simulink model "processor_with_peripherals"  (R2025a)
settings: Solver=FixedStepDiscrete  StartTime=0.0  StopTime=inf  RelTol=1e-3
libraries: simulink x6
(part 4 of 5)

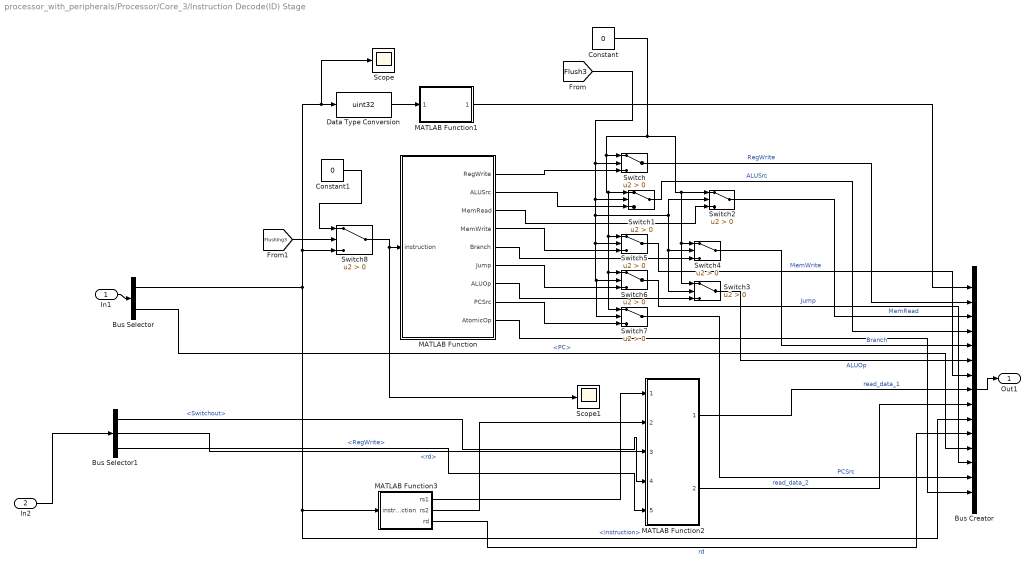
== system processor_with_peripherals/Processor/Core_3/Instruction Decode(ID) Stage ==
  In1 : Inport
  In2 : Inport  Port=2
  Bus Creator : BusCreator  Inputs=15  OutDataTypeStr=Bus: IDEX_Bus  NonVirtualBus=on
  Bus Selector : BusSelector  OutputSignals=Instruction,PC
  Bus Selector1 : BusSelector  OutputSignals=Switchout,rd,RegWrite
  Constant : Constant  Value=0  OutDataTypeStr=uint8
  Constant1 : Constant  Value=0
  Data Type Conversion : DataTypeConversion  OutDataTypeStr=uint32  SaturateOnIntegerOverflow=off  RndMeth=Floor
  MATLAB Function : MATLAB Function  TreatAsAtomicUnit=on
  MATLAB Function1 : MATLAB Function  TreatAsAtomicUnit=on
  MATLAB Function2 : MATLAB Function  TreatAsAtomicUnit=on
  MATLAB Function3 : MATLAB Function  TreatAsAtomicUnit=on
  Scope : Scope
      settings: ActiveDisplayYMinimum=-8.6059552101299882E+7  ActiveDisplayYMaximum=2.8669047582629967E+8  DataLoggingVariableName=ScopeData4
  Scope1 : Scope
      settings: ActiveDisplayYMinimum=-0.20992987297977578  ActiveDisplayYMaximum=4.3440753791982463  DataLoggingVariableName=ScopeData5
  Switch{,1..2,5..6} (5 alike) : Switch  Criteria=u2 > Threshold  OutDataTypeStr=boolean  SaturateOnIntegerOverflow=off  InputSameDT=off
  Switch3 : Switch  Criteria=u2 > Threshold  OutDataTypeStr=uint32  SaturateOnIntegerOverflow=off  InputSameDT=off
  Switch4 : Switch  Criteria=u2 > Threshold  OutDataTypeStr=uint32  SaturateOnIntegerOverflow=off  InputSameDT=off
  Switch7 : Switch  Criteria=u2 > Threshold  OutDataTypeStr=uint32  SaturateOnIntegerOverflow=off  InputSameDT=off
  Switch8 : Switch  Criteria=u2 > Threshold  SaturateOnIntegerOverflow=off  InputSameDT=off
  Out1 : Outport
  wires:
  Bus Creator/1 -> Out1/1
  In1/1 -> Bus Selector/1
  Bus Selector/1 -> Data Type Conversion/1, Scope/1, Switch8/3, MATLAB Function3/1(instruction), Bus Creator/10  "<Instruction>"
  MATLAB Function2/1(ReadData1) -> Bus Creator/8  "read_data_1"
  MATLAB Function2/2(ReadData2) -> Bus Creator/9  "read_data_2"
  MATLAB Function1/1(immediate_out) -> Bus Creator/1
  MATLAB Function3/3(rd) -> Bus Creator/11  "rd"
  MATLAB Function/7(ALUOp) -> Switch3/3
  MATLAB Function/6(Jump) -> Switch6/3
  MATLAB Function/5(Branch) -> Switch4/3
  MATLAB Function/4(MemWrite) -> Switch5/3
  MATLAB Function/3(MemRead) -> Switch2/3
  MATLAB Function/2(ALUSrc) -> Switch1/3
  Bus Selector1/2 -> MATLAB Function2/3(WriteAddr)  "<rd>"
  Bus Selector1/3 -> MATLAB Function2/5(WriteEnable)  "<RegWrite>"
  Bus Selector1/1 -> MATLAB Function2/4(WriteData)  "<Switchout>"
  MATLAB Function3/2(rs2) -> MATLAB Function2/2(ReadAddr2)
  Bus Selector/2 -> Bus Creator/12  "<PC>"
  MATLAB Function/8(PCSrc) -> Switch7/3
  MATLAB Function/1(RegWrite) -> Switch/3
  [Flush3] -> Switch1/2, Switch3/2, Switch4/2, Switch2/2, Switch7/2, Switch6/2, Switch5/2, Switch/2
  Constant/1 -> Switch3/1, Switch4/1, Switch2/1, Switch7/1, Switch6/1, Switch5/1, Switch1/1, Switch/1
  Switch/1 -> Bus Creator/2  "RegWrite"
  Switch2/1 -> Bus Creator/3  "MemRead"
  Switch1/1 -> Bus Creator/4  "ALUSrc"
  Switch4/1 -> Bus Creator/5  "Branch"
  Switch3/1 -> Bus Creator/6  "ALUOp"
  Switch5/1 -> Bus Creator/7  "MemWrite"
  Switch6/1 -> Bus Creator/13  "Jump"
  Switch7/1 -> Bus Creator/14  "PCSrc"
  MATLAB Function3/1(rs1) -> MATLAB Function2/1(ReadAddr1)
  In2/1 -> Bus Selector1/1
  Switch8/1 -> Scope1/1, MATLAB Function/1(instruction)
  Constant1/1 -> Switch8/1
  [Flushing3] -> Switch8/2
  Data Type Conversion/1 -> MATLAB Function1/1(instruction)
  MATLAB Function/9(AtomicOp) -> Bus Creator/15

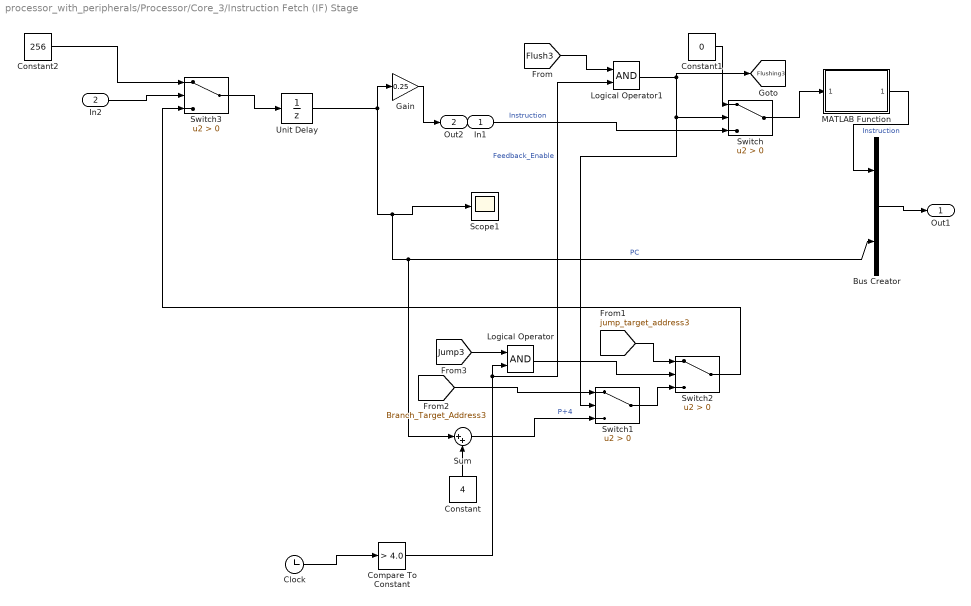
== system processor_with_peripherals/Processor/Core_3/Instruction Fetch (IF) Stage ==
  In1 : Inport
  In2 : Inport  Port=2
  Bus Creator : BusCreator  Inputs=2  OutDataTypeStr=Bus: IFID_Bus  NonVirtualBus=on
  Clock : Clock
  Compare To Constant : simulink/Logic and Bit Operations/Compare To Constant  relop=>  const=4.0  OutDataTypeStr=boolean
  Constant : Constant  Value=4
  Constant1 : Constant  Value=0
  Constant2 : Constant  Value=256  OutDataTypeStr=uint32
  Gain : Gain  Gain=0.25  OutDataTypeStr=uint32
  Logical Operator : Logic  AllPortsSameDT=off  OutDataTypeStr=boolean
  Logical Operator1 : Logic  AllPortsSameDT=off  OutDataTypeStr=boolean
  MATLAB Function : MATLAB Function  TreatAsAtomicUnit=on
  Scope1 : Scope
      settings: ActiveDisplayYMinimum=14.083038013644533  ActiveDisplayYMaximum=56.284353840527714  DataLoggingVariableName=ScopeData6
  Sum : Sum  Inputs=|++  OutDataTypeStr=uint32  AccumDataTypeStr=uint32
  Switch : Switch  Criteria=u2 > Threshold  OutDataTypeStr=uint32  SaturateOnIntegerOverflow=off  InputSameDT=off
  Switch1 : Switch  Criteria=u2 > Threshold  OutDataTypeStr=uint32  SaturateOnIntegerOverflow=off  InputSameDT=off
  Switch2 : Switch  Criteria=u2 > Threshold  OutDataTypeStr=uint32  SaturateOnIntegerOverflow=off  InputSameDT=off
  Switch3 : Switch  Criteria=u2 > Threshold  SaturateOnIntegerOverflow=off  InputSameDT=off
  Unit Delay : UnitDelay  HasFrameUpgradeWarning=on
  Out1 : Outport
  Out2 : Outport  Port=2
  tag scope: Flushing3=global
  wires:
  Unit Delay/1 -> Scope1/1, Bus Creator/2, Sum/1, Gain/1  "PC"
  Constant/1 -> Sum/2
  In1/1 -> Switch/3  "Instruction"
  [jump_target_address3] -> Switch2/1
  Logical Operator1/1 -> Switch/2, Switch1/2, [Flushing3]
  Sum/1 -> Switch1/3  "P+4"
  Bus Creator/1 -> Out1/1
  Switch1/1 -> Switch2/3
  Switch2/1 -> Switch3/3
  [Jump3] -> Logical Operator/1
  [Branch_Target_Address3] -> Switch1/1
  Clock/1 -> Compare To Constant/1
  Compare To Constant/1 -> Logical Operator1/2, Logical Operator/2  "Feedback_Enable"
  Logical Operator/1 -> Switch2/2
  [Flush3] -> Logical Operator1/1
  MATLAB Function/1(scalar_out) -> Bus Creator/1  "Instruction"
  Switch/1 -> MATLAB Function/1(vector_in)
  Constant1/1 -> Switch/1
  Gain/1 -> Out2/1
  Switch3/1 -> Unit Delay/1
  In2/1 -> Switch3/2
  Constant2/1 -> Switch3/1

== system processor_with_peripherals/Processor/Core_3/Memory Access ==
  In1 : Inport
  Bus Creator : BusCreator  Inputs=4  OutDataTypeStr=Bus: MEMWB_Bus
  Bus Selector : BusSelector  OutputSignals=read_data_2,ALU_Result,MemWrite,RegWrite,MemRead,rd,AtomicOp
  Switch : Switch  Criteria=u2 > Threshold  SaturateOnIntegerOverflow=off  InputSameDT=off
  Out1 : Outport
  Out2 : Outport  Port=2
  Out3 : Outport  Port=3
  Out4 : Outport  Port=4
  Out5 : Outport  Port=5
  wires:
  In1/1 -> Bus Selector/1
  Bus Selector/2 -> Switch/1, Out2/1, Bus Creator/1  "<ALU_Result>"
  Bus Selector/6 -> Bus Creator/4  "<rd>"
  Bus Selector/3 -> Out5/1  "<MemWrite>"
  Bus Selector/5 -> Bus Creator/3, Out4/1  "<MemRead>"
  Bus Selector/4 -> Bus Creator/2  "<RegWrite>"
  Bus Selector/1 -> Switch/3  "<read_data_2>"
  Bus Creator/1 -> Out1/1
  Switch/1 -> Out3/1
  Bus Selector/7 -> Switch/2  "<AtomicOp>"

== system processor_with_peripherals/Processor/Core_3/Write Back ==
  In1 : Inport
  In2 : Inport  Port=2
  Bus Creator : BusCreator  Inputs=3
  Bus Selector : BusSelector  OutputSignals=ALU_Result,rd,MemRead,RegWrite
  Switch : Switch  Criteria=u2 > Threshold  SaturateOnIntegerOverflow=off  InputSameDT=off
  Out1 : Outport
  wires:
  Bus Creator/1 -> Out1/1
  In1/1 -> Bus Selector/1
  Bus Selector/1 -> Switch/3  "<ALU_Result>"
  Bus Selector/2 -> Bus Creator/2  "<rd>"
  Bus Selector/4 -> Bus Creator/3  "<RegWrite>"
  Bus Selector/3 -> Switch/2  "<MemRead>"
  Switch/1 -> Bus Creator/1  "Switchout"
  In2/1 -> Switch/1

== matlab function processor_with_peripherals/Processor/Core_2/Execute (EX) Stage/MATLAB Function ==
  data: Operand1 input; ALU_Result output int32 size=1; Operand2 input; ALUOp input; Instruction input; Zero_Flag output boolean size=1; AtomicOp input
function [ALU_Result, Zero_Flag] = alu(Operand1, Operand2, ALUOp, Instruction, AtomicOp)
% This is the final ALU code, supporting standard operations and
% the RISC-V "A" extension for atomic memory operations.

    instr = uint32(Instruction);
    alu_op_val = ALUOp(1)*2 + ALUOp(2); 

    % Extract function fields
    funct3 = bitshift(bitand(instr, uint32(hex2dec('7000'))), -12);
    funct7 = bitshift(bitand(instr, uint32(hex2dec('FE000000'))), -25);
    funct5 = bitshift(bitand(instr, uint32(hex2dec('F8000000'))), -27); % For atomic ops

    ALU_Result = int32(0);

    if AtomicOp
        % --- This is an Atomic Operation ---
        switch funct5
            case 0,  ALU_Result = Operand1 + Operand2;  % AMOADD.W
            case 1,  ALU_Result = Operand2;            % AMOSWAP.W
            case 4,  ALU_Result = bitxor(Operand1, Operand2); % AMOXOR.W
            case 12, ALU_Result = bitand(Operand1, Operand2); % AMOAND.W
            case 20, ALU_Result = bitor(Operand1, Operand2);  % AMOOR.W
            otherwise, ALU_Result = Operand1;
        end
    else
        % --- This is a Normal Operation ---
        switch alu_op_val
            case 0 % For LW, SW, ADDI, JAL, etc.
                ALU_Result = Operand1 + Operand2;
            case 1 % For Branches
                ALU_Result = Operand1 - Operand2;
            case 2 % R-type instructions
                switch funct3
                    case 0 % ADD or SUB
                        if funct7 == 32, ALU_Result = Operand1 - Operand2; else, ALU_Result = Operand1 + Operand2; end
                    case 1, ALU_Result = int32(bitshift(uint32(Operand1), Operand2)); % SLL
                    case 2, if Operand1 < Operand2, ALU_Result = int32(1); else, ALU_Result = int32(0); end % SLT
                    case 4, ALU_Result = bitxor(Operand1, Operand2); % XOR
                    case 6, ALU_Result = bitor(Operand1, Operand2);  % OR
                    case 7, ALU_Result = bitand(Operand1, Operand2); % AND
                    otherwise, ALU_Result = int32(0);
                end
            case 3 % I-type instructions
                 switch funct3
                    case 0, ALU_Result = Operand1 + Operand2; % ADDI
                    case 2, if Operand1 < Operand2, ALU_Result = int32(1); else, ALU_Result = int32(0); end % SLTI
                    case 4, ALU_Result = bitxor(Operand1, Operand2); % XORI
                    case 6, ALU_Result = bitor(Operand1, Operand2);  % ORI
                    case 7, ALU_Result = bitand(Operand1, Operand2); % ANDI
                    otherwise, ALU_Result = int32(0);
                 end
        end
    end
    
    Zero_Flag = (ALU_Result == 0);
end

== matlab function processor_with_peripherals/Processor/Core_1/Instruction Decode(ID) Stage/MATLAB Function ==
  data: instruction input; RegWrite output; ALUSrc output; MemRead output; MemWrite output; Branch output; Jump output boolean; ALUOp output; PCSrc output; AtomicOp output
function [RegWrite, ALUSrc, MemRead, MemWrite, Branch, Jump, ALUOp, PCSrc, AtomicOp] = control_unit(instruction)
% This is the final Control Unit code. It takes an instruction and
% generates all necessary control signals for the datapath.

    instr = uint32(instruction);
    
    % --- Opcode Definitions ---
    OPCODE_R_TYPE   = uint32(hex2dec('33'));
    OPCODE_I_TYPE   = uint32(hex2dec('13'));
    OPCODE_LOAD     = uint32(hex2dec('03'));
    OPCODE_STORE    = uint32(hex2dec('23'));
    OPCODE_BRANCH   = uint32(hex2dec('63'));
    OPCODE_JAL      = uint32(hex2dec('6F'));
    OPCODE_JALR     = uint32(hex2dec('67'));
    OPCODE_LUI      = uint32(hex2dec('37'));
    OPCODE_AMO      = uint32(hex2dec('2F'));

    % --- Control Signal Initialization ---
    RegWrite = false; ALUSrc = false; MemRead = false; MemWrite = false;
    Branch = false; Jump = false; PCSrc = false; AtomicOp = false;
    ALUOp = [0 0];
    
    opcode = bitand(instr, uint32(127));

    % --- Decoder Logic ---
    switch opcode
        case OPCODE_R_TYPE
            RegWrite = true; ALUSrc = false; ALUOp = [1 0];
        case OPCODE_I_TYPE
            RegWrite = true; ALUSrc = true; ALUOp = [1 1];
        case OPCODE_LOAD
            RegWrite = true; ALUSrc = true; MemRead = true; ALUOp = [0 0];
        case OPCODE_STORE
            ALUSrc = true; MemWrite = true; ALUOp = [0 0];
        case OPCODE_BRANCH
            Branch = true; ALUSrc = false; ALUOp = [0 1];
        case OPCODE_JAL
            RegWrite = true; Jump = true; ALUSrc = true; PCSrc = true; ALUOp = [0 0];
        case OPCODE_JALR
            RegWrite = true; Jump = true; ALUSrc = true; ALUOp = [0 0];
        case OPCODE_LUI
            RegWrite = true; ALUSrc = true; PCSrc = true; ALUOp = [0 0];
        case OPCODE_AMO
            RegWrite = true; MemRead = true; MemWrite = true; AtomicOp = true; ALUOp = [1 0];
    end
end

== matlab function processor_with_peripherals/Processor/Core_1/Instruction Decode(ID) Stage/MATLAB Function1 ==
  data: instruction input uint32; immediate_out output int32
function immediate_out = immediate_generator(instruction)
% This function uses a robust subtraction method for sign extension
% to prevent all overflow errors in the Simulink Coder.

    instr = uint32(instruction);
    opcode = bitand(instr, uint32(127));

    % Define opcodes
    OPCODE_I_TYPE   = uint32(hex2dec('13'));
    OPCODE_LOAD     = uint32(hex2dec('03'));
    OPCODE_JALR     = uint32(hex2dec('67'));
    OPCODE_STORE    = uint32(hex2dec('23'));
    OPCODE_BRANCH   = uint32(hex2dec('63'));
    OPCODE_LUI      = uint32(hex2dec('37'));
    OPCODE_JAL      = uint32(hex2dec('6F'));

    imm_val = int32(0); % Use a signed integer for the final value
    
    switch opcode
        case {OPCODE_I_TYPE, OPCODE_LOAD, OPCODE_JALR} % I-type
            imm_unsigned = bitshift(instr, -20);
            sign_bit = bitget(imm_unsigned, 12);
            if sign_bit
                % Two's complement: val - 2^12
                imm_val = int32(imm_unsigned) - 4096; 
            else
                imm_val = int32(imm_unsigned);
            end

        case OPCODE_STORE % S-type
            imm_11_5 = bitshift(instr, -25);
            imm_4_0  = bitshift(bitand(instr, uint32(hex2dec('F80'))), -7);
            imm_unsigned = bitor(imm_11_5, imm_4_0);
            sign_bit = bitget(imm_unsigned, 12);
            if sign_bit
                imm_val = int32(imm_unsigned) - 4096;
            else
                imm_val = int32(imm_unsigned);
            end
            
        case OPCODE_BRANCH % B-type
            imm_12   = bitshift(bitand(instr, uint32(hex2dec('80000000'))), -19);
            imm_10_5 = bitshift(bitand(instr, uint32(hex2dec('7E000000'))), -20);
            imm_4_1  = bitshift(bitand(instr, uint32(hex2dec('F00'))), -7);
            imm_11   = bitshift(bitand(instr, uint32(hex2dec('80'))), 4);
            imm_unsigned = bitor(bitor(bitor(imm_12, imm_11), imm_10_5), imm_4_1);
            sign_bit = bitget(imm_unsigned, 13);
            if sign_bit
                imm_val = int32(imm_unsigned) - 8192; % 2^13
            else
                imm_val = int32(imm_unsigned);
            end
        
        case OPCODE_LUI % U-type -- THIS IS THE FIX --
            % For LUI, the immediate is the entire upper 20 bits.
            % The value is simply the instruction bits themselves, treated
            % as a 32-bit signed number. We cast the uint32 instruction
            % directly to int32, which correctly interprets the sign bit.
            imm_val = typecast(instr, 'int32');

        case OPCODE_JAL % J-type
            imm_20   = bitshift(bitand(instr, uint32(hex2dec('80000000'))), -11);
            imm_10_1 = bitshift(bitand(instr, uint32(hex2dec('7FE00000'))), -20);
            imm_11   = bitshift(bitand(instr, uint32(hex2dec('100000'))), -9);
            imm_19_12= bitand(instr, uint32(hex2dec('FF000')));
            imm_unsigned = bitor(bitor(bitor(imm_20, imm_19_12), imm_11), imm_10_1);
            sign_bit = bitget(imm_unsigned, 21);
            if sign_bit
                imm_val = int32(imm_unsigned) - 2097152; % 2^21
            else
                imm_val = int32(imm_unsigned);
            end
    end
    
    immediate_out = imm_val;
end

== matlab function processor_with_peripherals/Processor/Core_1/Instruction Decode(ID) Stage/MATLAB Function2 ==
  data: ReadAddr1 input; ReadData1 output int32; ReadAddr2 input; WriteAddr input; WriteData input; WriteEnable input; ReadData2 output int32
function [ReadData1, ReadData2] = register_file(ReadAddr1, ReadAddr2, WriteAddr, WriteData, WriteEnable)
% Implements a 32-register file for a RISC-V processor.
% x0 is hardwired to zero. Uses 1-based MATLAB indexing.

    persistent Registers;
    if isempty(Registers)
        Registers = zeros(32, 1, 'int32');
    end

    % 1. Handle the Write-Back from the WB stage first (synchronous write)
    if WriteEnable
        if WriteAddr > 0 % Do not write to register x0
            % MATLAB arrays are 1-based, so we add 1 to the 0-based RISC-V address
            Registers(WriteAddr + 1) = WriteData;
        end
    end

    % 2. Perform the Reads for the ID stage (combinational read)
    if ReadAddr1 == 0
        ReadData1 = int32(0);
    else
        ReadData1 = Registers(ReadAddr1 + 1);
    end

    if ReadAddr2 == 0
        ReadData2 = int32(0);
    else
        ReadData2 = Registers(ReadAddr2 + 1);
    end
end

== matlab function processor_with_peripherals/Processor/Core_1/Instruction Decode(ID) Stage/MATLAB Function3 ==
  data: instruction input; rs1 output uint8; rs2 output uint8; rd output uint8
function [rs1, rs2, rd] = bit_slicer(instruction)
% This function correctly extracts the rs1, rs2, and rd fields
% from a 32-bit RISC-V instruction word.

    instr = uint32(instruction);

    % Extract rd (destination register, bits 11:7)
    rd  = uint8(bitshift(bitand(instr, uint32(hex2dec('F80'))), -7));

    % Extract rs1 (source register 1, bits 19:15)
    rs1 = uint8(bitshift(bitand(instr, uint32(hex2dec('F8000'))), -15));

    % Extract rs2 (source register 2, bits 24:20)
    rs2 = uint8(bitshift(bitand(instr, uint32(hex2dec('1F00000'))), -20));
end

== matlab function processor_with_peripherals/Processor/Core_1/Instruction Fetch (IF) Stage/MATLAB Function ==
  data: vector_in input; scalar_out output uint32
function scalar_out = to_scalar(vector_in)
% This function extracts the first element from an input vector
% and ensures the output is a uint32 scalar.
    scalar_out = uint32(vector_in(1));
end

== matlab function processor_with_peripherals/Processor/Core_2/Instruction Decode(ID) Stage/MATLAB Function ==
  data: instruction input; RegWrite output; ALUSrc output; MemRead output; MemWrite output; Branch output; Jump output boolean; ALUOp output; PCSrc output; AtomicOp output
function [RegWrite, ALUSrc, MemRead, MemWrite, Branch, Jump, ALUOp, PCSrc, AtomicOp] = control_unit(instruction)
% This is the final Control Unit code. It takes an instruction and
% generates all necessary control signals for the datapath.

    instr = uint32(instruction);
    
    % --- Opcode Definitions ---
    OPCODE_R_TYPE   = uint32(hex2dec('33'));
    OPCODE_I_TYPE   = uint32(hex2dec('13'));
    OPCODE_LOAD     = uint32(hex2dec('03'));
    OPCODE_STORE    = uint32(hex2dec('23'));
    OPCODE_BRANCH   = uint32(hex2dec('63'));
    OPCODE_JAL      = uint32(hex2dec('6F'));
    OPCODE_JALR     = uint32(hex2dec('67'));
    OPCODE_LUI      = uint32(hex2dec('37'));
    OPCODE_AMO      = uint32(hex2dec('2F'));

    % --- Control Signal Initialization ---
    RegWrite = false; ALUSrc = false; MemRead = false; MemWrite = false;
    Branch = false; Jump = false; PCSrc = false; AtomicOp = false;
    ALUOp = [0 0];
    
    opcode = bitand(instr, uint32(127));

    % --- Decoder Logic ---
    switch opcode
        case OPCODE_R_TYPE
            RegWrite = true; ALUSrc = false; ALUOp = [1 0];
        case OPCODE_I_TYPE
            RegWrite = true; ALUSrc = true; ALUOp = [1 1];
        case OPCODE_LOAD
            RegWrite = true; ALUSrc = true; MemRead = true; ALUOp = [0 0];
        case OPCODE_STORE
            ALUSrc = true; MemWrite = true; ALUOp = [0 0];
        case OPCODE_BRANCH
            Branch = true; ALUSrc = false; ALUOp = [0 1];
        case OPCODE_JAL
            RegWrite = true; Jump = true; ALUSrc = true; PCSrc = true; ALUOp = [0 0];
        case OPCODE_JALR
            RegWrite = true; Jump = true; ALUSrc = true; ALUOp = [0 0];
        case OPCODE_LUI
            RegWrite = true; ALUSrc = true; PCSrc = true; ALUOp = [0 0];
        case OPCODE_AMO
            RegWrite = true; MemRead = true; MemWrite = true; AtomicOp = true; ALUOp = [1 0];
    end
end

== matlab function processor_with_peripherals/Processor/Core_2/Instruction Decode(ID) Stage/MATLAB Function1 ==
  data: instruction input uint32; immediate_out output int32
function immediate_out = immediate_generator(instruction)
% This function uses a robust subtraction method for sign extension
% to prevent all overflow errors in the Simulink Coder.

    instr = uint32(instruction);
    opcode = bitand(instr, uint32(127));

    % Define opcodes
    OPCODE_I_TYPE   = uint32(hex2dec('13'));
    OPCODE_LOAD     = uint32(hex2dec('03'));
    OPCODE_JALR     = uint32(hex2dec('67'));
    OPCODE_STORE    = uint32(hex2dec('23'));
    OPCODE_BRANCH   = uint32(hex2dec('63'));
    OPCODE_LUI      = uint32(hex2dec('37'));
    OPCODE_JAL      = uint32(hex2dec('6F'));

    imm_val = int32(0); % Use a signed integer for the final value
    
    switch opcode
        case {OPCODE_I_TYPE, OPCODE_LOAD, OPCODE_JALR} % I-type
            imm_unsigned = bitshift(instr, -20);
            sign_bit = bitget(imm_unsigned, 12);
            if sign_bit
                % Two's complement: val - 2^12
                imm_val = int32(imm_unsigned) - 4096; 
            else
                imm_val = int32(imm_unsigned);
            end

        case OPCODE_STORE % S-type
            imm_11_5 = bitshift(instr, -25);
            imm_4_0  = bitshift(bitand(instr, uint32(hex2dec('F80'))), -7);
            imm_unsigned = bitor(imm_11_5, imm_4_0);
            sign_bit = bitget(imm_unsigned, 12);
            if sign_bit
                imm_val = int32(imm_unsigned) - 4096;
            else
                imm_val = int32(imm_unsigned);
            end
            
        case OPCODE_BRANCH % B-type
            imm_12   = bitshift(bitand(instr, uint32(hex2dec('80000000'))), -19);
            imm_10_5 = bitshift(bitand(instr, uint32(hex2dec('7E000000'))), -20);
            imm_4_1  = bitshift(bitand(instr, uint32(hex2dec('F00'))), -7);
            imm_11   = bitshift(bitand(instr, uint32(hex2dec('80'))), 4);
            imm_unsigned = bitor(bitor(bitor(imm_12, imm_11), imm_10_5), imm_4_1);
            sign_bit = bitget(imm_unsigned, 13);
            if sign_bit
                imm_val = int32(imm_unsigned) - 8192; % 2^13
            else
                imm_val = int32(imm_unsigned);
            end
        
        case OPCODE_LUI % U-type -- THIS IS THE FIX --
            % For LUI, the immediate is the entire upper 20 bits.
            % The value is simply the instruction bits themselves, treated
            % as a 32-bit signed number. We cast the uint32 instruction
            % directly to int32, which correctly interprets the sign bit.
            imm_val = typecast(instr, 'int32');

        case OPCODE_JAL % J-type
            imm_20   = bitshift(bitand(instr, uint32(hex2dec('80000000'))), -11);
            imm_10_1 = bitshift(bitand(instr, uint32(hex2dec('7FE00000'))), -20);
            imm_11   = bitshift(bitand(instr, uint32(hex2dec('100000'))), -9);
            imm_19_12= bitand(instr, uint32(hex2dec('FF000')));
            imm_unsigned = bitor(bitor(bitor(imm_20, imm_19_12), imm_11), imm_10_1);
            sign_bit = bitget(imm_unsigned, 21);
            if sign_bit
                imm_val = int32(imm_unsigned) - 2097152; % 2^21
            else
                imm_val = int32(imm_unsigned);
            end
    end
    
    immediate_out = imm_val;
end

== matlab function processor_with_peripherals/Processor/Core_2/Instruction Decode(ID) Stage/MATLAB Function2 ==
  data: ReadAddr1 input; ReadData1 output int32; ReadAddr2 input; WriteAddr input; WriteData input; WriteEnable input; ReadData2 output int32
function [ReadData1, ReadData2] = register_file(ReadAddr1, ReadAddr2, WriteAddr, WriteData, WriteEnable)
% Implements a 32-register file for a RISC-V processor.
% x0 is hardwired to zero. Uses 1-based MATLAB indexing.

    persistent Registers;
    if isempty(Registers)
        Registers = zeros(32, 1, 'int32');
    end

    % 1. Handle the Write-Back from the WB stage first (synchronous write)
    if WriteEnable
        if WriteAddr > 0 % Do not write to register x0
            % MATLAB arrays are 1-based, so we add 1 to the 0-based RISC-V address
            Registers(WriteAddr + 1) = WriteData;
        end
    end

    % 2. Perform the Reads for the ID stage (combinational read)
    if ReadAddr1 == 0
        ReadData1 = int32(0);
    else
        ReadData1 = Registers(ReadAddr1 + 1);
    end

    if ReadAddr2 == 0
        ReadData2 = int32(0);
    else
        ReadData2 = Registers(ReadAddr2 + 1);
    end
end

== matlab function processor_with_peripherals/Processor/Core_2/Instruction Decode(ID) Stage/MATLAB Function3 ==
  data: instruction input; rs1 output uint8; rs2 output uint8; rd output uint8
function [rs1, rs2, rd] = bit_slicer(instruction)
% This function correctly extracts the rs1, rs2, and rd fields
% from a 32-bit RISC-V instruction word.

    instr = uint32(instruction);

    % Extract rd (destination register, bits 11:7)
    rd  = uint8(bitshift(bitand(instr, uint32(hex2dec('F80'))), -7));

    % Extract rs1 (source register 1, bits 19:15)
    rs1 = uint8(bitshift(bitand(instr, uint32(hex2dec('F8000'))), -15));

    % Extract rs2 (source register 2, bits 24:20)
    rs2 = uint8(bitshift(bitand(instr, uint32(hex2dec('1F00000'))), -20));
end

== matlab function processor_with_peripherals/Processor/Core_2/Instruction Fetch (IF) Stage/MATLAB Function ==
  data: vector_in input; scalar_out output uint32
function scalar_out = to_scalar(vector_in)
% This function extracts the first element from an input vector
% and ensures the output is a uint32 scalar.
    scalar_out = uint32(vector_in(1));
end

== matlab function processor_with_peripherals/Processor/Core_3/Execute (EX) Stage/MATLAB Function ==
  data: Operand1 input; ALU_Result output int32 size=1; Operand2 input; ALUOp input; Instruction input; Zero_Flag output boolean size=1; AtomicOp input
function [ALU_Result, Zero_Flag] = alu(Operand1, Operand2, ALUOp, Instruction, AtomicOp)
% This is the final ALU code, supporting standard operations and
% the RISC-V "A" extension for atomic memory operations.

    instr = uint32(Instruction);
    alu_op_val = ALUOp(1)*2 + ALUOp(2); 

    % Extract function fields
    funct3 = bitshift(bitand(instr, uint32(hex2dec('7000'))), -12);
    funct7 = bitshift(bitand(instr, uint32(hex2dec('FE000000'))), -25);
    funct5 = bitshift(bitand(instr, uint32(hex2dec('F8000000'))), -27); % For atomic ops

    ALU_Result = int32(0);

    if AtomicOp
        % --- This is an Atomic Operation ---
        switch funct5
            case 0,  ALU_Result = Operand1 + Operand2;  % AMOADD.W
            case 1,  ALU_Result = Operand2;            % AMOSWAP.W
            case 4,  ALU_Result = bitxor(Operand1, Operand2); % AMOXOR.W
            case 12, ALU_Result = bitand(Operand1, Operand2); % AMOAND.W
            case 20, ALU_Result = bitor(Operand1, Operand2);  % AMOOR.W
            otherwise, ALU_Result = Operand1;
        end
    else
        % --- This is a Normal Operation ---
        switch alu_op_val
            case 0 % For LW, SW, ADDI, JAL, etc.
                ALU_Result = Operand1 + Operand2;
            case 1 % For Branches
                ALU_Result = Operand1 - Operand2;
            case 2 % R-type instructions
                switch funct3
                    case 0 % ADD or SUB
                        if funct7 == 32, ALU_Result = Operand1 - Operand2; else, ALU_Result = Operand1 + Operand2; end
                    case 1, ALU_Result = int32(bitshift(uint32(Operand1), Operand2)); % SLL
                    case 2, if Operand1 < Operand2, ALU_Result = int32(1); else, ALU_Result = int32(0); end % SLT
                    case 4, ALU_Result = bitxor(Operand1, Operand2); % XOR
                    case 6, ALU_Result = bitor(Operand1, Operand2);  % OR
                    case 7, ALU_Result = bitand(Operand1, Operand2); % AND
                    otherwise, ALU_Result = int32(0);
                end
            case 3 % I-type instructions
                 switch funct3
                    case 0, ALU_Result = Operand1 + Operand2; % ADDI
                    case 2, if Operand1 < Operand2, ALU_Result = int32(1); else, ALU_Result = int32(0); end % SLTI
                    case 4, ALU_Result = bitxor(Operand1, Operand2); % XORI
                    case 6, ALU_Result = bitor(Operand1, Operand2);  % ORI
                    case 7, ALU_Result = bitand(Operand1, Operand2); % ANDI
                    otherwise, ALU_Result = int32(0);
                 end
        end
    end
    
    Zero_Flag = (ALU_Result == 0);
end

== matlab function processor_with_peripherals/Processor/Core_3/Instruction Decode(ID) Stage/MATLAB Function ==
  data: instruction input; RegWrite output; ALUSrc output; MemRead output; MemWrite output; Branch output; Jump output; ALUOp output; PCSrc output; AtomicOp output
function [RegWrite, ALUSrc, MemRead, MemWrite, Branch, Jump, ALUOp, PCSrc, AtomicOp] = control_unit(instruction)
% This is the final Control Unit code. It takes an instruction and
% generates all necessary control signals for the datapath.

    instr = uint32(instruction);
    
    % --- Opcode Definitions ---
    OPCODE_R_TYPE   = uint32(hex2dec('33'));
    OPCODE_I_TYPE   = uint32(hex2dec('13'));
    OPCODE_LOAD     = uint32(hex2dec('03'));
    OPCODE_STORE    = uint32(hex2dec('23'));
    OPCODE_BRANCH   = uint32(hex2dec('63'));
    OPCODE_JAL      = uint32(hex2dec('6F'));
    OPCODE_JALR     = uint32(hex2dec('67'));
    OPCODE_LUI      = uint32(hex2dec('37'));
    OPCODE_AMO      = uint32(hex2dec('2F'));

    % --- Control Signal Initialization ---
    RegWrite = false; ALUSrc = false; MemRead = false; MemWrite = false;
    Branch = false; Jump = false; PCSrc = false; AtomicOp = false;
    ALUOp = [0 0];
    
    opcode = bitand(instr, uint32(127));

    % --- Decoder Logic ---
    switch opcode
        case OPCODE_R_TYPE
            RegWrite = true; ALUSrc = false; ALUOp = [1 0];
        case OPCODE_I_TYPE
            RegWrite = true; ALUSrc = true; ALUOp = [1 1];
        case OPCODE_LOAD
            RegWrite = true; ALUSrc = true; MemRead = true; ALUOp = [0 0];
        case OPCODE_STORE
            ALUSrc = true; MemWrite = true; ALUOp = [0 0];
        case OPCODE_BRANCH
            Branch = true; ALUSrc = false; ALUOp = [0 1];
        case OPCODE_JAL
            RegWrite = true; Jump = true; ALUSrc = true; PCSrc = true; ALUOp = [0 0];
        case OPCODE_JALR
            RegWrite = true; Jump = true; ALUSrc = true; ALUOp = [0 0];
        case OPCODE_LUI
            RegWrite = true; ALUSrc = true; PCSrc = true; ALUOp = [0 0];
        case OPCODE_AMO
            RegWrite = true; MemRead = true; MemWrite = true; AtomicOp = true; ALUOp = [1 0];
    end
end

== matlab function processor_with_peripherals/Processor/Core_3/Instruction Decode(ID) Stage/MATLAB Function1 ==
  data: instruction input uint32; immediate_out output int32
function immediate_out = immediate_generator(instruction)
% This function uses a robust subtraction method for sign extension
% to prevent all overflow errors in the Simulink Coder.

    instr = uint32(instruction);
    opcode = bitand(instr, uint32(127));

    % Define opcodes
    OPCODE_I_TYPE   = uint32(hex2dec('13'));
    OPCODE_LOAD     = uint32(hex2dec('03'));
    OPCODE_JALR     = uint32(hex2dec('67'));
    OPCODE_STORE    = uint32(hex2dec('23'));
    OPCODE_BRANCH   = uint32(hex2dec('63'));
    OPCODE_LUI      = uint32(hex2dec('37'));
    OPCODE_JAL      = uint32(hex2dec('6F'));

    imm_val = int32(0); % Use a signed integer for the final value
    
    switch opcode
        case {OPCODE_I_TYPE, OPCODE_LOAD, OPCODE_JALR} % I-type
            imm_unsigned = bitshift(instr, -20);
            sign_bit = bitget(imm_unsigned, 12);
            if sign_bit
                % Two's complement: val - 2^12
                imm_val = int32(imm_unsigned) - 4096; 
            else
                imm_val = int32(imm_unsigned);
            end

        case OPCODE_STORE % S-type
            imm_11_5 = bitshift(instr, -25);
            imm_4_0  = bitshift(bitand(instr, uint32(hex2dec('F80'))), -7);
            imm_unsigned = bitor(imm_11_5, imm_4_0);
            sign_bit = bitget(imm_unsigned, 12);
            if sign_bit
                imm_val = int32(imm_unsigned) - 4096;
            else
                imm_val = int32(imm_unsigned);
            end
            
        case OPCODE_BRANCH % B-type
            imm_12   = bitshift(bitand(instr, uint32(hex2dec('80000000'))), -19);
            imm_10_5 = bitshift(bitand(instr, uint32(hex2dec('7E000000'))), -20);
            imm_4_1  = bitshift(bitand(instr, uint32(hex2dec('F00'))), -7);
            imm_11   = bitshift(bitand(instr, uint32(hex2dec('80'))), 4);
            imm_unsigned = bitor(bitor(bitor(imm_12, imm_11), imm_10_5), imm_4_1);
            sign_bit = bitget(imm_unsigned, 13);
            if sign_bit
                imm_val = int32(imm_unsigned) - 8192; % 2^13
            else
                imm_val = int32(imm_unsigned);
            end
        
        case OPCODE_LUI % U-type -- THIS IS THE FIX --
            % For LUI, the immediate is the entire upper 20 bits.
            % The value is simply the instruction bits themselves, treated
            % as a 32-bit signed number. We cast the uint32 instruction
            % directly to int32, which correctly interprets the sign bit.
            imm_val = typecast(instr, 'int32');

        case OPCODE_JAL % J-type
            imm_20   = bitshift(bitand(instr, uint32(hex2dec('80000000'))), -11);
            imm_10_1 = bitshift(bitand(instr, uint32(hex2dec('7FE00000'))), -20);
            imm_11   = bitshift(bitand(instr, uint32(hex2dec('100000'))), -9);
            imm_19_12= bitand(instr, uint32(hex2dec('FF000')));
            imm_unsigned = bitor(bitor(bitor(imm_20, imm_19_12), imm_11), imm_10_1);
            sign_bit = bitget(imm_unsigned, 21);
            if sign_bit
                imm_val = int32(imm_unsigned) - 2097152; % 2^21
            else
                imm_val = int32(imm_unsigned);
            end
    end
    
    immediate_out = imm_val;
end

== matlab function processor_with_peripherals/Processor/Core_3/Instruction Decode(ID) Stage/MATLAB Function2 ==
  data: ReadAddr1 input; ReadData1 output int32; ReadAddr2 input; WriteAddr input; WriteData input; WriteEnable input; ReadData2 output int32
function [ReadData1, ReadData2] = register_file(ReadAddr1, ReadAddr2, WriteAddr, WriteData, WriteEnable)
% Implements a 32-register file for a RISC-V processor.
% x0 is hardwired to zero. Uses 1-based MATLAB indexing.

    persistent Registers;
    if isempty(Registers)
        Registers = zeros(32, 1, 'int32');
    end

    % 1. Handle the Write-Back from the WB stage first (synchronous write)
    if WriteEnable
        if WriteAddr > 0 % Do not write to register x0
            % MATLAB arrays are 1-based, so we add 1 to the 0-based RISC-V address
            Registers(WriteAddr + 1) = WriteData;
        end
    end

    % 2. Perform the Reads for the ID stage (combinational read)
    if ReadAddr1 == 0
        ReadData1 = int32(0);
    else
        ReadData1 = Registers(ReadAddr1 + 1);
    end

    if ReadAddr2 == 0
        ReadData2 = int32(0);
    else
        ReadData2 = Registers(ReadAddr2 + 1);
    end
end

== matlab function processor_with_peripherals/Processor/Core_3/Instruction Decode(ID) Stage/MATLAB Function3 ==
  data: instruction input; rs1 output uint8; rs2 output uint8; rd output uint8
function [rs1, rs2, rd] = bit_slicer(instruction)
% This function correctly extracts the rs1, rs2, and rd fields
% from a 32-bit RISC-V instruction word.

    instr = uint32(instruction);

    % Extract rd (destination register, bits 11:7)
    rd  = uint8(bitshift(bitand(instr, uint32(hex2dec('F80'))), -7));

    % Extract rs1 (source register 1, bits 19:15)
    rs1 = uint8(bitshift(bitand(instr, uint32(hex2dec('F8000'))), -15));

    % Extract rs2 (source register 2, bits 24:20)
    rs2 = uint8(bitshift(bitand(instr, uint32(hex2dec('1F00000'))), -20));
end

== matlab function processor_with_peripherals/Processor/Core_3/Instruction Fetch (IF) Stage/MATLAB Function ==
  data: vector_in input; scalar_out output uint32
function scalar_out = to_scalar(vector_in)
% This function extracts the first element from an input vector
% and ensures the output is a uint32 scalar.
    scalar_out = uint32(vector_in(1));
end

== matlab function processor_with_peripherals/Processor/Common hardware/MATLAB Function ==
  data: Addr_0 input; Mem_RData_0 output; WData_0 input; MemRead_0 input; MemWrite_0 input; Addr_1 input; WData_1 input; MemRead_1 input; MemWrite_1 input; Addr_2 input; WData_2 input; MemRead_2 input; MemWrite_2 input; Addr_3 input; WData_3 input; MemRead_3 input; MemWrite_3 input; Mem_RData_from_RAM input; Mem_RData_1 output; Mem_RData_2 output; Mem_RData_3 output; RAM_Addr output; RAM_WData output; RAM_MemRead output; RAM_MemWrite output
function [Mem_RData_0, Mem_RData_1, Mem_RData_2, Mem_RData_3, RAM_Addr, RAM_WData, RAM_MemRead, RAM_MemWrite] = Bus_Arbiter_4_Core( ...
    Addr_0, WData_0, MemRead_0, MemWrite_0, ...
    Addr_1, WData_1, MemRead_1, MemWrite_1, ...
    Addr_2, WData_2, MemRead_2, MemWrite_2, ...
    Addr_3, WData_3, MemRead_3, MemWrite_3, ...
    Mem_RData_from_RAM)
% This function implements a fair, round-robin bus arbiter for a 4-core system.

    persistent last_grant;
    if isempty(last_grant)
        last_grant = 3; % Initialize to 3, so Core 0 gets the first chance.
    end

    % Default outputs
    RAM_Addr = int32(0);
    RAM_WData = int32(0);
    RAM_MemRead = false;
    RAM_MemWrite = false;
    Mem_RData_0 = int32(0);
    Mem_RData_1 = int32(0);
    Mem_RData_2 = int32(0);
    Mem_RData_3 = int32(0);
    
    % Gather all requests into arrays for easier processing
    requests = [ (MemRead_0 || MemWrite_0), (MemRead_1 || MemWrite_1), (MemRead_2 || MemWrite_2), (MemRead_3 || MemWrite_3) ];
    
    % --- Round-Robin Arbitration Logic ---
    % Check each core for a request, starting from the one after the last grant.
    for i = 1:4
        core_idx = mod(last_grant + i, 4); % Cycles through 0, 1, 2, 3
        
        if requests(core_idx + 1) % MATLAB arrays are 1-based
            % Grant access to this core
            switch core_idx
                case 0
                    RAM_Addr = Addr_0; RAM_WData = WData_0; RAM_MemRead = MemRead_0; RAM_MemWrite = MemWrite_0;
                    Mem_RData_0 = Mem_RData_from_RAM;
                case 1
                    RAM_Addr = Addr_1; RAM_WData = WData_1; RAM_MemRead = MemRead_1; RAM_MemWrite = MemWrite_1;
                    Mem_RData_1 = Mem_RData_from_RAM;
                case 2
                    RAM_Addr = Addr_2; RAM_WData = WData_2; RAM_MemRead = MemRead_2; RAM_MemWrite = MemWrite_2;
                    Mem_RData_2 = Mem_RData_from_RAM;
                case 3
                    RAM_Addr = Addr_3; RAM_WData = WData_3; RAM_MemRead = MemRead_3; RAM_MemWrite = MemWrite_3;
                    Mem_RData_3 = Mem_RData_from_RAM;
            end
            
            last_grant = core_idx; % Remember who got the grant
            return; % Exit the function once a grant is given
        end
    end
end

== matlab function processor_with_peripherals/Processor/Common hardware/MATLAB Function1 ==
  data: Address input int32; WriteData input; MemRead input; MemWrite input; ReadData output int32
function ReadData = Shared_Data_Memory(Address, WriteData, MemRead, MemWrite)
% This function models a synchronous shared data memory that only
% performs a read or write when explicitly enabled.

    persistent Memory;
    MEMORY_SIZE_WORDS = 16384; % The size of our memory
    
    if isempty(Memory)
        % Initialize a 64KB memory space
        Memory = zeros(MEMORY_SIZE_WORDS, 1, 'int32');
    end

    % Default output is 0. This value is used if no read occurs.
    ReadData = int32(0);
    
    % --- Address Range and Control Signal Check ---
    % Only proceed if the address is valid AND a read or write is requested.
    if (Address >= 0 && Address < (MEMORY_SIZE_WORDS * 4))
    
        % Convert the byte address to a 1-based word index.
        wordAddress = (Address / 4) + 1;

        % --- NEW: Conditional Read ---
        % Perform the read operation only if MemRead is true.
        if MemRead
            ReadData = Memory(wordAddress);
        end

        % Perform the write operation only if MemWrite is true.
        if MemWrite
            Memory(wordAddress) = WriteData;
        end
    end
    % If the address is out of range or no read/write signal is active,
    % the function correctly does nothing and outputs 0.
end

== matlab function processor_with_peripherals/Processor/Core_0/Instruction Decode(ID) Stage/MATLAB Function1 ==
  data: instruction input uint32; immediate_out output int32
function immediate_out = immediate_generator(instruction)
% This function uses a robust subtraction method for sign extension
% to prevent all overflow errors in the Simulink Coder.

    instr = uint32(instruction);
    opcode = bitand(instr, uint32(127));

    % Define opcodes
    OPCODE_I_TYPE   = uint32(hex2dec('13'));
    OPCODE_LOAD     = uint32(hex2dec('03'));
    OPCODE_JALR     = uint32(hex2dec('67'));
    OPCODE_STORE    = uint32(hex2dec('23'));
    OPCODE_BRANCH   = uint32(hex2dec('63'));
    OPCODE_LUI      = uint32(hex2dec('37'));
    OPCODE_JAL      = uint32(hex2dec('6F'));

    imm_val = int32(0); % Use a signed integer for the final value
    
    switch opcode
        case {OPCODE_I_TYPE, OPCODE_LOAD, OPCODE_JALR} % I-type
            imm_unsigned = bitshift(instr, -20);
            sign_bit = bitget(imm_unsigned, 12);
            if sign_bit
                % Two's complement: val - 2^12
                imm_val = int32(imm_unsigned) - 4096; 
            else
                imm_val = int32(imm_unsigned);
            end

        case OPCODE_STORE % S-type
            imm_11_5 = bitshift(instr, -25);
            imm_4_0  = bitshift(bitand(instr, uint32(hex2dec('F80'))), -7);
            imm_unsigned = bitor(imm_11_5, imm_4_0);
            sign_bit = bitget(imm_unsigned, 12);
            if sign_bit
                imm_val = int32(imm_unsigned) - 4096;
            else
                imm_val = int32(imm_unsigned);
            end
            
        case OPCODE_BRANCH % B-type
            imm_12   = bitshift(bitand(instr, uint32(hex2dec('80000000'))), -19);
            imm_10_5 = bitshift(bitand(instr, uint32(hex2dec('7E000000'))), -20);
            imm_4_1  = bitshift(bitand(instr, uint32(hex2dec('F00'))), -7);
            imm_11   = bitshift(bitand(instr, uint32(hex2dec('80'))), 4);
            imm_unsigned = bitor(bitor(bitor(imm_12, imm_11), imm_10_5), imm_4_1);
            sign_bit = bitget(imm_unsigned, 13);
            if sign_bit
                imm_val = int32(imm_unsigned) - 8192; % 2^13
            else
                imm_val = int32(imm_unsigned);
            end
        
        case OPCODE_LUI % U-type -- THIS IS THE FIX --
            % For LUI, the immediate is the entire upper 20 bits.
            % The value is simply the instruction bits themselves, treated
            % as a 32-bit signed number. We cast the uint32 instruction
            % directly to int32, which correctly interprets the sign bit.
            imm_val = typecast(instr, 'int32');

        case OPCODE_JAL % J-type
            imm_20   = bitshift(bitand(instr, uint32(hex2dec('80000000'))), -11);
            imm_10_1 = bitshift(bitand(instr, uint32(hex2dec('7FE00000'))), -20);
            imm_11   = bitshift(bitand(instr, uint32(hex2dec('100000'))), -9);
            imm_19_12= bitand(instr, uint32(hex2dec('FF000')));
            imm_unsigned = bitor(bitor(bitor(imm_20, imm_19_12), imm_11), imm_10_1);
            sign_bit = bitget(imm_unsigned, 21);
            if sign_bit
                imm_val = int32(imm_unsigned) - 2097152; % 2^21
            else
                imm_val = int32(imm_unsigned);
            end
    end
    
    immediate_out = imm_val;
end

== matlab function processor_with_peripherals/Processor/Common hardware/MATLAB Function2 ==
  data: Address input; IRQ_0 output; MemWrite input; IRQ_1 output; IRQ_2 output; IRQ_3 output
function [IRQ_0, IRQ_1, IRQ_2, IRQ_3] = IPI_Controller_4_Core(Address, MemWrite)
% This block models an Inter-Processor Interrupt controller for a 4-core system.

    % Define four unique, high-memory addresses for the IPI registers
    IPI_ADDR_0 = 4294901760; % 0xFFFF0000
    IPI_ADDR_1 = 4294901764; % 0xFFFF0004
    IPI_ADDR_2 = 4294901768; % 0xFFFF0008
    IPI_ADDR_3 = 4294901772; % 0xFFFF000C

    % Default outputs are inactive
    IRQ_0 = false;
    IRQ_1 = false;
    IRQ_2 = false;
    IRQ_3 = false;

    % Check for a write to one of the IPI addresses
    if MemWrite
        if Address == IPI_ADDR_0
            IRQ_0 = true;
        elseif Address == IPI_ADDR_1
            IRQ_1 = true;
        elseif Address == IPI_ADDR_2
            IRQ_2 = true;
        elseif Address == IPI_ADDR_3
            IRQ_3 = true;
        end
    end
end

== matlab function processor_with_peripherals/MATLAB Function ==
  data: Address input; WriteData input; MemWrite input
function UART_TX(Address, WriteData, MemWrite)
% This function models a simple memory-mapped UART transmitter
% for printf-style debugging.

    % Define the unique memory-mapped address for the UART Tx register
    UART_TX_ADDR = 4294967284; % 0xFFFFFFF4
    
    % Check if a core is performing a write to our address
    if MemWrite && (Address == UART_TX_ADDR)
        % The processor wrote to our transmit register.
        % Print the character to the MATLAB command window.
        fprintf('%c', char(WriteData));
    end
end

== matlab function processor_with_peripherals/Processor/Core_0/Instruction Decode(ID) Stage/MATLAB Function ==
  data: instruction input; RegWrite output; ALUSrc output; MemRead output; MemWrite output; Branch output; Jump output boolean; ALUOp output; PCSrc output; AtomicOp output
function [RegWrite, ALUSrc, MemRead, MemWrite, Branch, Jump, ALUOp, PCSrc, AtomicOp] = control_unit(instruction)
% This is the final Control Unit code. It takes an instruction and
% generates all necessary control signals for the datapath.

    instr = uint32(instruction);
    
    % --- Opcode Definitions ---
    OPCODE_R_TYPE   = uint32(hex2dec('33'));
    OPCODE_I_TYPE   = uint32(hex2dec('13'));
    OPCODE_LOAD     = uint32(hex2dec('03'));
    OPCODE_STORE    = uint32(hex2dec('23'));
    OPCODE_BRANCH   = uint32(hex2dec('63'));
    OPCODE_JAL      = uint32(hex2dec('6F'));
    OPCODE_JALR     = uint32(hex2dec('67'));
    OPCODE_LUI      = uint32(hex2dec('37'));
    OPCODE_AMO      = uint32(hex2dec('2F'));

    % --- Control Signal Initialization ---
    RegWrite = false; ALUSrc = false; MemRead = false; MemWrite = false;
    Branch = false; Jump = false; PCSrc = false; AtomicOp = false;
    ALUOp = [0 0];
    
    opcode = bitand(instr, uint32(127));

    % --- Decoder Logic ---
    switch opcode
        case OPCODE_R_TYPE
            RegWrite = true; ALUSrc = false; ALUOp = [1 0];
        case OPCODE_I_TYPE
            RegWrite = true; ALUSrc = true; ALUOp = [1 1];
        case OPCODE_LOAD
            RegWrite = true; ALUSrc = true; MemRead = true; ALUOp = [0 0];
        case OPCODE_STORE
            ALUSrc = true; MemWrite = true; ALUOp = [0 0];
        case OPCODE_BRANCH
            Branch = true; ALUSrc = false; ALUOp = [0 1];
        case OPCODE_JAL
            RegWrite = true; Jump = true; ALUSrc = true; PCSrc = true; ALUOp = [0 0];
        case OPCODE_JALR
            RegWrite = true; Jump = true; ALUSrc = true; ALUOp = [0 0];
        case OPCODE_LUI
            RegWrite = true; ALUSrc = true; PCSrc = true; ALUOp = [0 0];
        case OPCODE_AMO
            RegWrite = true; MemRead = true; MemWrite = true; AtomicOp = true; ALUOp = [1 0];
    end
end
